simulink model "Balancing_Logic"  (R2020a)
settings: configuration reference "BMS_Sw_CodeGenConfig" (kept outside this file)
values from neighbouring files (symbols this model uses):
  BalNotActWait = 30    [DD_Balancing_Logic.sldd]
  BalOffWait = 20    [DD_Balancing_Logic.sldd]
  BalOnWait = 60    [DD_Balancing_Logic.sldd]
  flgEnBalancing = 1    [DD_Balancing_Logic.sldd]
  TargetDeltaV = 0.01    [DD_Balancing_Logic.sldd]
undefined symbols (not defined in the file or in its folder): Ns_Module, NumModules
settings Model: DataDictionary=DD_Balancing_Logic.sldd  ExtModeTrigDuration=5  Creator=cpatel  LastModifiedBy=cpatel
settings ConfigSetRef: SourceName=BMS_Sw_CodeGenConfig

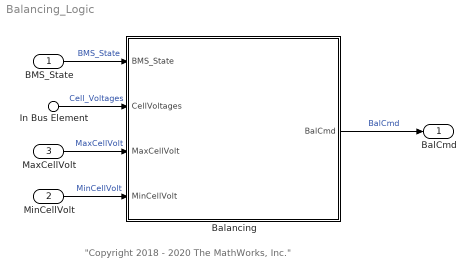
== system Balancing_Logic ==
  note: "Copyright 2018 - 2020 The MathWorks, Inc."
  BMS_State : Inport  OutDataTypeStr=Enum: BMS_State_Enum  PortDimensions=1  SampleTime=[5,0]
  MinCellVolt : Inport  Port=2  OutDataTypeStr=single  PortDimensions=1  SampleTime=[5,0]
  MaxCellVolt : Inport  Port=3  OutDataTypeStr=single  PortDimensions=1  SampleTime=[5,0]
  In Bus Element : Inport  Port=4  PortName=BMS_Input  Element=Cell_Voltages
  Balancing : Stateflow chart  TreatAsAtomicUnit=on  VariantControl=(default)
  BalCmd : Outport  OutDataTypeStr=boolean  PortDimensions=[1,NumModules*Ns_Module]  SampleTime=[5,0]  VectorParamsAs1DForOutWhenUnconnected=off
  wires:
  Balancing/1(BalCmd) -> BalCmd/1  "BalCmd"
  BMS_State/1 -> Balancing/1(BMS_State)  "BMS_State"
  MinCellVolt/1 -> Balancing/4(MinCellVolt)  "MinCellVolt"
  MaxCellVolt/1 -> Balancing/3(MaxCellVolt)  "MaxCellVolt"
  In Bus Element/1 -> Balancing/2(CellVoltages)  "Cell_Voltages"

== stateflow chart Balancing_Logic/Balancing ==
  state BalancingOFF
    en:
    BalCmd(:,:) = false;
    en,du:
    DeltaCellVolt = MaxCellVolt - MinCellVolt;
  state BalancingON
    en, du:
    DeltaCellVolt = MaxCellVolt - MinCellVolt;
    state BalActive
      en, du:
      BalCmd = ((CellVoltages - MinCellVolt) > TargetDeltaV/2)';
      flgBalCompl = all(~BalCmd);
    state BalNotActive
    (default) -> BalActive
    BalNotActive -> BalActive [order 1] : [after(BalNotActWait,sec) && ...
        | DeltaCellVolt > TargetDeltaV]
    BalActive -> BalNotActive : [flgBalCompl]
  note: "Copyright 2018 - 2019 The MathWorks, Inc."
  (default) -> BalancingOFF : {flgBalCompl = true;}
  BalancingOFF -> BalancingON : [flgEnBalancing && ...
      | BMS_State ~= BMS_State_Enum.BMS_Driving && ...
      | after(BalOffWait,sec) && ...
      | DeltaCellVolt > TargetDeltaV]
  BalancingON -> BalancingOFF : [BMS_State == BMS_State_Enum.BMS_Driving] %In Driving State
  BalNotActive -> BalancingOFF [order 2] : [after(BalOnWait,sec)]
  data: BMS_State input Enum: BMS_State_Enum; CellVoltages input single; TargetDeltaV parameter; BalCmd output boolean size=[1,Ns_Module*NumModules] =boolean(zeros(1,Ns_Module*NumModules)); flgBalCompl local; MaxCellVolt input single; MinCellVolt input single; BalNotActWait parameter; BalOffWait parameter; BalOnWait parameter; flgEnBalancing parameter; DeltaCellVolt local single =single(0)
